simulink model "Double_Damper"  (R2018b)
settings: Solver=VariableStepAuto  StartTime=0.0  StopTime=10.0  RelTol=1e-3  EnableMultiTasking=on
libraries: dspinverses x1
settings Model: Creator=student  LastModifiedBy=Федор
settings OptimizationCC: OptimizeBlockIOStorage=off  BufferReuse=off  GlobalBufferReuse=off  ExpressionFolding=off  LocalBlockOutputs=off  LifeSpan=inf  OptimizeDataStoreBuffers=off  BusAssignmentInplaceUpdate=off
settings DebuggingCC: SFUnexpectedBacktrackingDiag=warning  SFNoUnconditionalDefaultTransitionDiag=warning
settings SFSimCC: SimUseLocalCustomCode=off
settings RTWCC: RTWUseLocalCustomCode=off
settings CodeAppCC: StateflowObjectComments=on  MATLABSourceComments=on
settings GRTTargetCC: TargetLangStandard=C89/C90 (ANSI)  GeneratePreprocessorConditionals=Disable all
settings ConfigComp: CovMetricSettings=dw  CovHtmlReporting=on  CovSaveCumulativeToWorkspaceVar=on  CovSaveSingleToWorkspaceVar=on  CovExternalEMLEnable=off

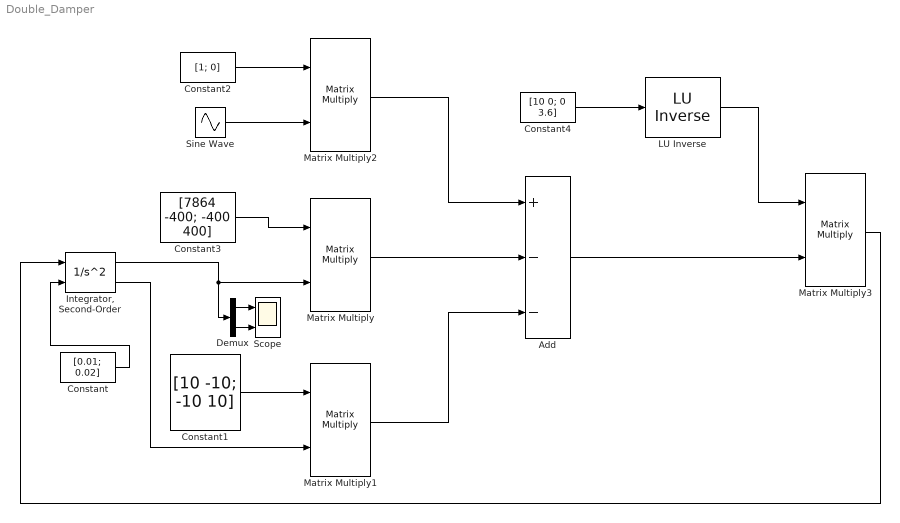
== system Double_Damper ==
  " LU Inverse" : dspinverses/ LU Inverse
      settings: SourceProductName=DSP System Toolbox
  Add : Sum  Inputs=+--
  Constant : Constant  Value=[0.01; 0.02]
  Constant1 : Constant  Value=[10 -10; -10 10]
  Constant2 : Constant  Value=[1; 0]
  Constant3 : Constant  Value=[7864 -400; -400 400]
  Constant4 : Constant  Value=[10 0; 0 3.6]
  Demux : Demux  Outputs=2
  "Integrator, Second-Order" : SecondOrderIntegrator  ICSourceDXDT=external
  Matrix Multiply{,1..3} (4 alike) : Product  Multiplication=Matrix(*)
  Scope : Scope  NumInputPorts=2
  Sine Wave : Sin  SampleTime=0
  wires:
  "Integrator, Second-Order"/2 -> Matrix Multiply1/2
  Constant3/1 -> Matrix Multiply/1
  Constant1/1 -> Matrix Multiply1/1
  Matrix Multiply/1 -> Add/2
  Matrix Multiply2/1 -> Add/1
  Matrix Multiply1/1 -> Add/3
  Constant4/1 -> " LU Inverse"/1
  Add/1 -> Matrix Multiply3/2
  " LU Inverse"/1 -> Matrix Multiply3/1
  Matrix Multiply3/1 -> "Integrator, Second-Order"/1
  Demux/2 -> Scope/2
  Demux/1 -> Scope/1
  "Integrator, Second-Order"/1 -> Demux/1, Matrix Multiply/2
  Constant2/1 -> Matrix Multiply2/1
  Sine Wave/1 -> Matrix Multiply2/2
  Constant/1 -> "Integrator, Second-Order"/2
